simulink model "Zika_Model_continous"  (R2022b)
settings: Solver=ode4  StartTime=0.0  StopTime=275  FixedStep=0.01  RelTol=1e-3
values from neighbouring files (symbols this model uses):
  A_b_0 = 0    [Cibernetica_project.m]
  A_w_0 = 0    [Cibernetica_project.m]
  E_b_0 = 0    [Cibernetica_project.m]
  E_v_0 = 0    [Cibernetica_project.m]
  E_w_0 = 0    [Cibernetica_project.m]
  I_b_0 = 1    [Cibernetica_project.m]
  I_bm_0 = 0    [Cibernetica_project.m]
  I_v_0 = 1    [Cibernetica_project.m]
  I_w_0 = 1    [Cibernetica_project.m]
  I_wm_0 = 0    [Cibernetica_project.m]
  P = [alpha, rho_b, rho_w, beta_w, sigma_w, gamma_w, mu_w, pi_b, beta_b,      sigma_b, gamma_b, mu_b, pi_v, beta_v, b_v, sigma_v, mu_v, p, eta,      q_a, q_r, q_i, r]    [Cibernetica_project.m]
  R_b_0 = 0    [Cibernetica_project.m]
  R_w_0 = 0    [Cibernetica_project.m]
  S_b_0 = 8000    [Cibernetica_project.m]
  S_v_0 = 0.225*10^6    (= 225000)    [Cibernetica_project.m]
  S_w_0 = 8000    [Cibernetica_project.m]
settings Model: Creator=anton  LastModifiedBy=angel
settings SolverCC: EnableFixedStepZeroCrossing=on  MaxZcPerStep=10

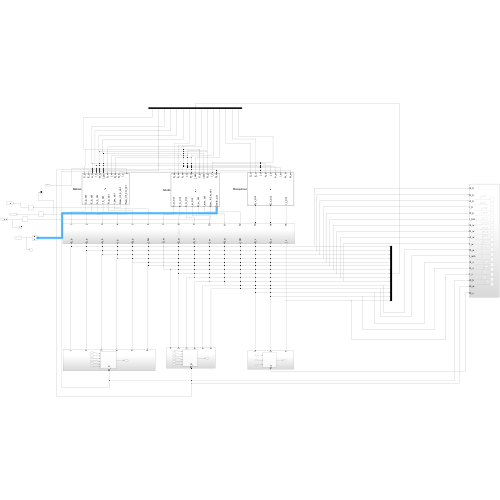
[thumbnail: Simulink's stored preview of the top-level diagram]
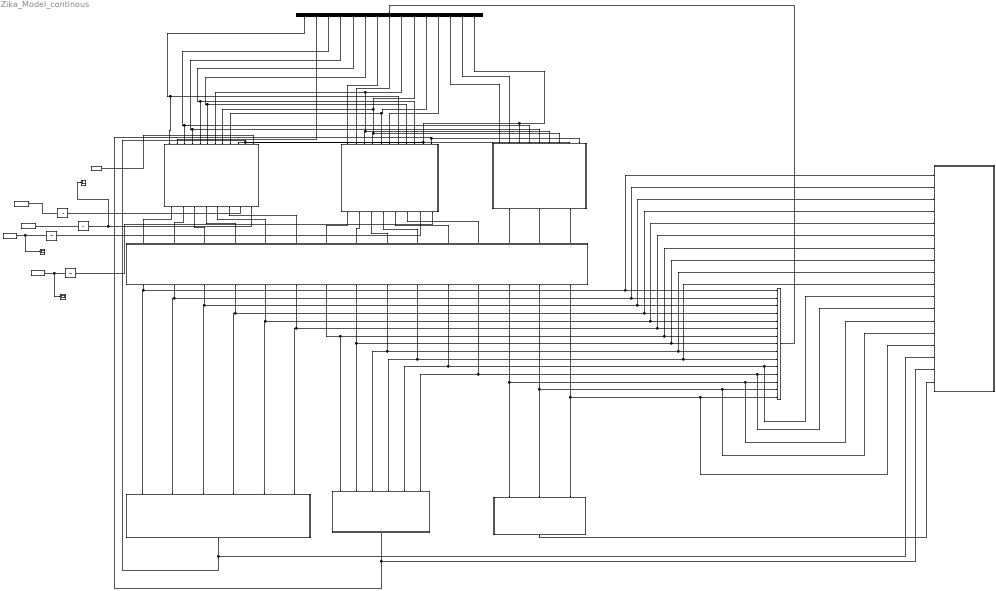
== system Zika_Model_continous ==
  Adults : MATLAB Function  TreatAsAtomicUnit=on  mask{P=P}
      mask prompts: P "Parametri del sistema"
  Babies : MATLAB Function  TreatAsAtomicUnit=on  mask{P=P}
      mask prompts: P "Parametri del sistema"
  Demux : Demux  Outputs=15
  Digital Clock : DigitalClock
  Integrator{,1..3} (4 alike) : Integrator
  Mosquitoes : MATLAB Function  TreatAsAtomicUnit=on  mask{P=P}
      mask prompts: P "Parametri del sistema"
  Mux : Mux  Inputs=15
  Scope : Scope
  Scope1 : Scope
  Scope2 : Scope
  Subsystem : Subsystem
  Subsystem1 : Subsystem
  Subsystem2 : Subsystem
  Subsystem3 : Subsystem
  Subsystem4 : Subsystem
  To Workspace : ToWorkspace  VariableName=New_inf_b  SampleTime=1
  To Workspace1 : ToWorkspace  VariableName=New_inf_w  SampleTime=1
  To Workspace2 : ToWorkspace  VariableName=New_inf_bm  SampleTime=1
  To Workspace3 : ToWorkspace  VariableName=Dead_Zika  SampleTime=1
  wires:
  Demux/5 -> Adults/9(R_b), Babies/5(R_b)
  Demux/6 -> Adults/8(I_bm), Babies/6(I_bm)
  Demux/9 -> Babies/7(A_w), Adults/3(A_w), Mosquitoes/6(A_w)
  Demux/4 -> Mosquitoes/5(I_b), Babies/4(I_b)
  Demux/7 -> Adults/1(S_w)
  Demux/2 -> Babies/2(E_b)
  Demux/11 -> Adults/5(R_w), Babies/9(R_w)
  Demux/15 -> Mosquitoes/3(I_v), Adults/10(I_v), Babies/11(I_v)
  Demux/14 -> Mosquitoes/2(E_v)
  Demux/8 -> Adults/2(E_w)
  Demux/13 -> Mosquitoes/1(S_v)
  Demux/10 -> Babies/8(I_w), Adults/4(I_w), Mosquitoes/7(I_w)
  Demux/12 -> Adults/6(I_wm)
  Subsystem2/1(N_v) -> Subsystem4/18(N_v)
  Demux/3 -> Mosquitoes/4(A_b), Babies/3(A_b)
  Demux/1 -> Babies/1(S_b), Adults/7(S_b)
  Mux/1 -> Demux/1
  Babies/1(S_b_dot) -> Subsystem3/1(In1)
  Babies/2(E_b_dot) -> Subsystem3/2(In2)
  Babies/3(A_b_dot) -> Subsystem3/3(In3)
  Babies/4(I_b_dot) -> Subsystem3/4(In4)
  Babies/5(R_b_dot) -> Subsystem3/5(In5)
  Babies/6(I_bm_dot) -> Subsystem3/6(In6)
  Adults/1(S_w_dot) -> Subsystem3/7(In7)
  Adults/2(E_w_dot) -> Subsystem3/8(In8)
  Adults/3(A_w_dot) -> Subsystem3/9(In9)
  Adults/4(I_w_dot) -> Subsystem3/10(In10)
  Adults/5(R_w_dot) -> Subsystem3/11(In11)
  Adults/6(I_wm_dot) -> Subsystem3/12(In12)
  Mosquitoes/1(S_v_dot) -> Subsystem3/13(In13)
  Mosquitoes/2(E_v_dot) -> Subsystem3/14(In14)
  Mosquitoes/3(I_v_dot) -> Subsystem3/15(In15)
  Subsystem3/1(S_b) -> Subsystem4/1(S_b), Mux/1, Subsystem/1(In1)
  Subsystem3/2(E_b) -> Subsystem4/2(E_b), Mux/2, Subsystem/2(In2)
  Subsystem3/3(A_b) -> Subsystem4/3(A_b), Mux/3, Subsystem/3(In3)
  Subsystem3/4(I_b) -> Subsystem4/4(I_b), Mux/4, Subsystem/4(In4)
  Subsystem3/5(R_b) -> Subsystem4/5(R_b), Mux/5, Subsystem/5(In5)
  Subsystem3/6(I_bm) -> Subsystem4/6(I_bm), Mux/6, Subsystem/6(In6)
  Subsystem3/7(S_w) -> Subsystem4/7(S_w), Mux/7, Subsystem1/1(In1)
  Subsystem3/8(E_w) -> Subsystem1/2(In2), Subsystem4/8(E_w), Mux/8
  Subsystem3/9(A_w) -> Subsystem1/3(In3), Subsystem4/9(A_w), Mux/9
  Subsystem3/10(I_w) -> Subsystem4/10(I_w), Mux/10, Subsystem1/4(In4)
  Subsystem3/11(R_w) -> Subsystem1/5(In5), Mux/11, Subsystem4/11(R_w)
  Subsystem3/12(I_wm) -> Subsystem4/12(I_wm), Mux/12, Subsystem1/6(In6)
  Subsystem3/13(S_v) -> Subsystem4/13(S_v), Mux/13, Subsystem2/1(In1)
  Subsystem3/15(I_v) -> Subsystem4/15(I_v), Mux/15, Subsystem2/3(In3)
  Subsystem3/14(E_v) -> Subsystem2/2(In2), Subsystem4/14(E_v), Mux/14
  Subsystem/1(N_b) -> Subsystem4/16(N_b), Mosquitoes/8(N_b), Babies/10(N_b)
  Subsystem1/1(N_w) -> Subsystem4/17(N_w), Mosquitoes/9(N_w), Adults/11(N_w)
  Babies/7(New_inf_b_dot) -> Integrator/1
  Integrator/1 -> To Workspace/1
  Integrator1/1 -> Scope1/1, To Workspace1/1
  Adults/7(New_Inf_w_dot) -> Integrator1/1
  Integrator2/1 -> To Workspace2/1
  Babies/8(New_inf_bm_dot) -> Scope/1, Integrator2/1
  Digital Clock/1 -> Babies/12(t)
  Integrator3/1 -> Scope2/1, To Workspace3/1
  Adults/8(Death_dot) -> Integrator3/1

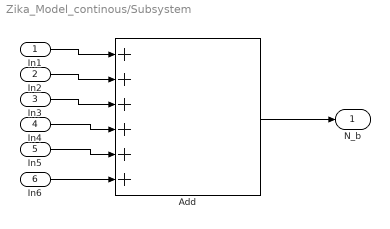
== system Zika_Model_continous/Subsystem ==
  In1 : Inport
  In2 : Inport  Port=2
  In3 : Inport  Port=3
  In4 : Inport  Port=4
  In5 : Inport  Port=5
  In6 : Inport  Port=6
  Add : Sum  Inputs=++++++
  N_b : Outport
  wires:
  In2/1 -> Add/2
  Add/1 -> N_b/1
  In1/1 -> Add/1
  In6/1 -> Add/6
  In5/1 -> Add/5
  In4/1 -> Add/4
  In3/1 -> Add/3

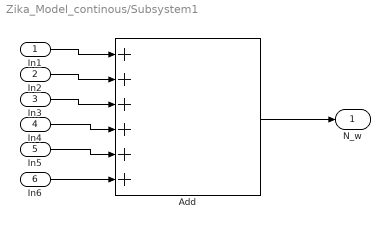
== system Zika_Model_continous/Subsystem1 ==
  In1 : Inport
  In2 : Inport  Port=2
  In3 : Inport  Port=3
  In4 : Inport  Port=4
  In5 : Inport  Port=5
  In6 : Inport  Port=6
  Add : Sum  Inputs=++++++
  N_w : Outport
  wires:
  In2/1 -> Add/2
  Add/1 -> N_w/1
  In1/1 -> Add/1
  In6/1 -> Add/6
  In5/1 -> Add/5
  In4/1 -> Add/4
  In3/1 -> Add/3

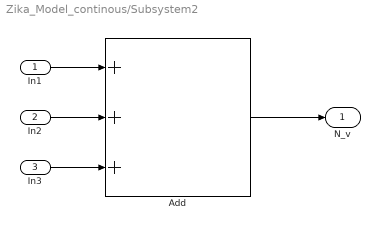
== system Zika_Model_continous/Subsystem2 ==
  In1 : Inport
  In2 : Inport  Port=2
  In3 : Inport  Port=3
  Add : Sum  Inputs=+++
  N_v : Outport
  wires:
  In2/1 -> Add/2
  Add/1 -> N_v/1
  In1/1 -> Add/1
  In3/1 -> Add/3

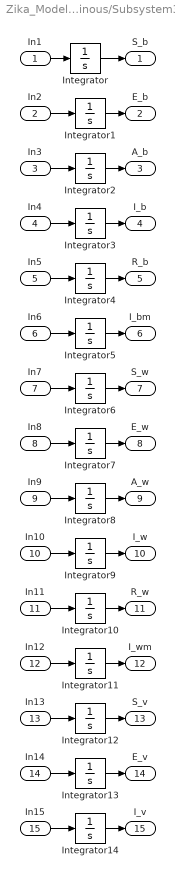
== system Zika_Model_continous/Subsystem3 ==
  In1 : Inport
  In2 : Inport  Port=2
  In3 : Inport  Port=3
  In4 : Inport  Port=4
  In5 : Inport  Port=5
  In6 : Inport  Port=6
  In7 : Inport  Port=7
  In8 : Inport  Port=8
  In9 : Inport  Port=9
  In10 : Inport  Port=10
  In11 : Inport  Port=11
  In12 : Inport  Port=12
  In13 : Inport  Port=13
  In14 : Inport  Port=14
  In15 : Inport  Port=15
  Integrator : Integrator  InitialCondition=S_b_0  ContinuousStateAttributes='S_b'
  Integrator1 : Integrator  InitialCondition=E_b_0  ContinuousStateAttributes='E_b'
  Integrator10 : Integrator  InitialCondition=R_w_0  ContinuousStateAttributes='R_w'
  Integrator11 : Integrator  InitialCondition=I_wm_0  ContinuousStateAttributes='I_wm'
  Integrator12 : Integrator  InitialCondition=S_v_0  ContinuousStateAttributes='S_v'
  Integrator13 : Integrator  InitialCondition=E_v_0  ContinuousStateAttributes='E_v'
  Integrator14 : Integrator  InitialCondition=I_v_0  ContinuousStateAttributes='I_v'
  Integrator2 : Integrator  InitialCondition=A_b_0  ContinuousStateAttributes='A_b'
  Integrator3 : Integrator  InitialCondition=I_b_0  ContinuousStateAttributes='I_b'
  Integrator4 : Integrator  InitialCondition=R_b_0  ContinuousStateAttributes='R_b'
  Integrator5 : Integrator  InitialCondition=I_bm_0  ContinuousStateAttributes='I_bm'
  Integrator6 : Integrator  InitialCondition=S_w_0  ContinuousStateAttributes='S_w'
  Integrator7 : Integrator  InitialCondition=E_w_0  ContinuousStateAttributes='E_w'
  Integrator8 : Integrator  InitialCondition=A_w_0  ContinuousStateAttributes='A_w'
  Integrator9 : Integrator  InitialCondition=I_w_0  ContinuousStateAttributes='I_w'
  S_b : Outport
  E_b : Outport  Port=2
  A_b : Outport  Port=3
  I_b : Outport  Port=4
  R_b : Outport  Port=5
  I_bm : Outport  Port=6
  S_w : Outport  Port=7
  E_w : Outport  Port=8
  A_w : Outport  Port=9
  I_w : Outport  Port=10
  R_w : Outport  Port=11
  I_wm : Outport  Port=12
  S_v : Outport  Port=13
  E_v : Outport  Port=14
  I_v : Outport  Port=15
  wires:
  In9/1 -> Integrator8/1
  In1/1 -> Integrator/1
  In12/1 -> Integrator11/1
  Integrator/1 -> S_b/1
  In2/1 -> Integrator1/1
  Integrator12/1 -> S_v/1
  Integrator13/1 -> E_v/1
  In13/1 -> Integrator12/1
  Integrator2/1 -> A_b/1
  Integrator1/1 -> E_b/1
  In6/1 -> Integrator5/1
  In14/1 -> Integrator13/1
  Integrator9/1 -> I_w/1
  Integrator4/1 -> R_b/1
  In11/1 -> Integrator10/1
  In3/1 -> Integrator2/1
  Integrator5/1 -> I_bm/1
  Integrator11/1 -> I_wm/1
  Integrator7/1 -> E_w/1
  Integrator14/1 -> I_v/1
  Integrator10/1 -> R_w/1
  In4/1 -> Integrator3/1
  Integrator3/1 -> I_b/1
  Integrator6/1 -> S_w/1
  In15/1 -> Integrator14/1
  Integrator8/1 -> A_w/1
  In10/1 -> Integrator9/1
  In5/1 -> Integrator4/1
  In7/1 -> Integrator6/1
  In8/1 -> Integrator7/1

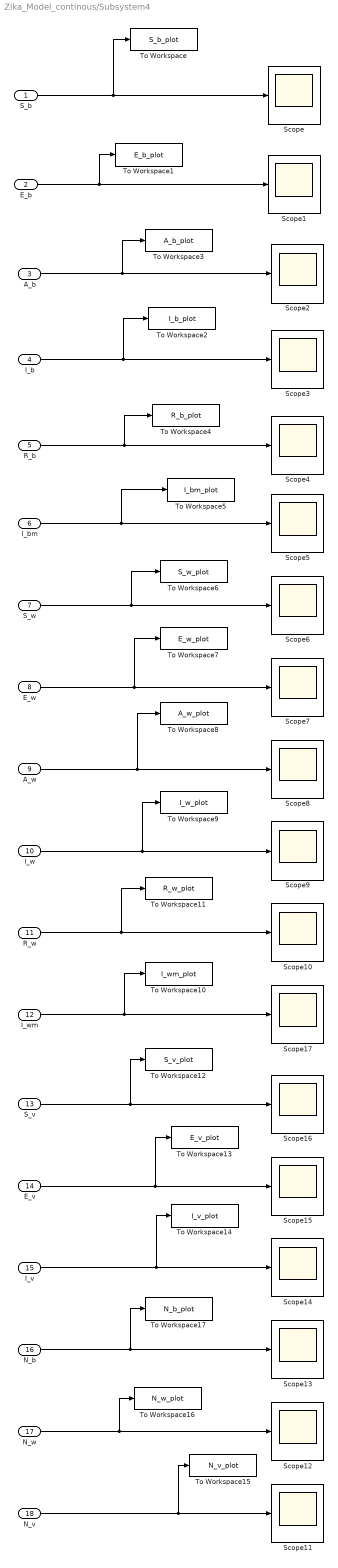
== system Zika_Model_continous/Subsystem4 ==
  S_b : Inport
  E_b : Inport  Port=2
  A_b : Inport  Port=3
  I_b : Inport  Port=4
  R_b : Inport  Port=5
  I_bm : Inport  Port=6
  S_w : Inport  Port=7
  E_w : Inport  Port=8
  A_w : Inport  Port=9
  I_w : Inport  Port=10
  R_w : Inport  Port=11
  I_wm : Inport  Port=12
  S_v : Inport  Port=13
  E_v : Inport  Port=14
  I_v : Inport  Port=15
  N_b : Inport  Port=16
  N_w : Inport  Port=17
  N_v : Inport  Port=18
  Scope{,1..17} (18 alike) : Scope
  To Workspace : ToWorkspace  VariableName=S_b_plot  SampleTime=1
  To Workspace1 : ToWorkspace  VariableName=E_b_plot  SampleTime=1
  To Workspace10 : ToWorkspace  VariableName=I_wm_plot  SampleTime=1
  To Workspace11 : ToWorkspace  VariableName=R_w_plot  SampleTime=1
  To Workspace12 : ToWorkspace  VariableName=S_v_plot  SampleTime=1
  To Workspace13 : ToWorkspace  VariableName=E_v_plot  SampleTime=1
  To Workspace14 : ToWorkspace  VariableName=I_v_plot  SampleTime=1
  To Workspace15 : ToWorkspace  VariableName=N_v_plot  SampleTime=1
  To Workspace16 : ToWorkspace  VariableName=N_w_plot  SampleTime=1
  To Workspace17 : ToWorkspace  VariableName=N_b_plot  SampleTime=1
  To Workspace2 : ToWorkspace  VariableName=I_b_plot  SampleTime=1
  To Workspace3 : ToWorkspace  VariableName=A_b_plot  SampleTime=1
  To Workspace4 : ToWorkspace  VariableName=R_b_plot  SampleTime=1
  To Workspace5 : ToWorkspace  VariableName=I_bm_plot  SampleTime=1
  To Workspace6 : ToWorkspace  VariableName=S_w_plot  SampleTime=1
  To Workspace7 : ToWorkspace  VariableName=E_w_plot  SampleTime=1
  To Workspace8 : ToWorkspace  VariableName=A_w_plot  SampleTime=1
  To Workspace9 : ToWorkspace  VariableName=I_w_plot  SampleTime=1
  wires:
  E_w/1 -> To Workspace7/1, Scope7/1
  E_b/1 -> To Workspace1/1, Scope1/1
  R_w/1 -> To Workspace11/1, Scope10/1
  A_b/1 -> To Workspace3/1, Scope2/1
  A_w/1 -> To Workspace8/1, Scope8/1
  R_b/1 -> To Workspace4/1, Scope4/1
  I_w/1 -> To Workspace9/1, Scope9/1
  S_v/1 -> To Workspace12/1, Scope16/1
  S_b/1 -> To Workspace/1, Scope/1
  I_wm/1 -> To Workspace10/1, Scope17/1
  I_bm/1 -> To Workspace5/1, Scope5/1
  I_b/1 -> To Workspace2/1, Scope3/1
  S_w/1 -> To Workspace6/1, Scope6/1
  E_v/1 -> To Workspace13/1, Scope15/1
  I_v/1 -> To Workspace14/1, Scope14/1
  N_v/1 -> To Workspace15/1, Scope11/1
  N_w/1 -> To Workspace16/1, Scope12/1
  N_b/1 -> To Workspace17/1, Scope13/1

== matlab function Zika_Model_continous/Adults ==
  data: S_w input; E_w input; A_w input; I_w input; R_w input; I_wm input; S_b input; S_w_dot output; I_bm input; R_b input; I_v input; N_w input; E_w_dot output; A_w_dot output; I_w_dot output; R_w_dot output; I_wm_dot output; P parameter; New_Inf_w_dot output; Death_dot output
function [S_w_dot, E_w_dot, A_w_dot, I_w_dot, R_w_dot, I_wm_dot, New_Inf_w_dot, Death_dot] = Adults(S_w,...
    E_w, A_w, I_w, R_w, I_wm, S_b, I_bm, R_b, I_v, N_w, P)

alpha = P(1);
rho_b = P(2);
rho_w = P(3);
beta_w = P(4);
sigma_w = P(5);
gamma_w = P(6);
mu_w = P(7);
pi_b = P(8);
beta_b = P(9);
sigma_b =  P(10);
gamma_b = P(11);
mu_b =  P(12);
pi_v =  P(13);
beta_v = P(14);
b_v = P(15);
sigma_v = P(16);
mu_v = P(17);
p = P(18);
eta = P(19);
q_a = P(20);
q_r = P(21);
q_i = P(22);
r = P(23);


lambda_w = (beta_w*b_v*I_v)/N_w;

S_w_dot = alpha*S_b - lambda_w*S_w - mu_w*S_w;
E_w_dot = lambda_w*S_w - (sigma_w + mu_v)*E_w;
A_w_dot = (1-p)*sigma_w*E_w - (gamma_w + mu_w)*A_w;
I_w_dot = p*sigma_w*E_w - (gamma_w + mu_w)*I_w;
I_wm_dot = alpha*I_bm - mu_w*I_wm;
R_w_dot = alpha*R_b + gamma_w*A_w + gamma_w*I_w - mu_w*R_w;

New_Inf_w_dot = sigma_w*E_w;
Death_dot = mu_w*(S_w + E_w + I_w + I_wm + R_w);

== matlab function Zika_Model_continous/Babies ==
  data: S_b input; S_b_dot output; E_b input; A_b input; I_b input; R_b input; I_bm input; E_b_dot output; A_b_dot output; I_b_dot output; R_b_dot output; I_bm_dot output; A_w input; I_w input; R_w input; P parameter; N_b input; I_v input; New_inf_b_dot output; New_inf_bm_dot output; t input
function [S_b_dot, E_b_dot, A_b_dot, I_b_dot, R_b_dot, I_bm_dot,New_inf_b_dot, New_inf_bm_dot] = Babies( ... 
    S_b, E_b, A_b, I_b, R_b, I_bm, A_w, I_w, R_w, P, N_b, I_v,t)
alpha = P(1);
rho_b = P(2);
rho_w = P(3);
beta_w = P(4);
sigma_w = P(5);
gamma_w = P(6);
mu_w = P(7);
pi_b = P(8);
beta_b = P(9);
sigma_b =  P(10);
gamma_b = P(11);
mu_b =  P(12);
pi_v =  P(13);
beta_v = P(14);
b_v = P(15);
sigma_v = P(16);
mu_v = P(17);
p = P(18);
eta = P(19);
q_a = P(20);
q_r = P(21);
q_i = P(22);
r = P(23);

if S_b > 0
    is_notzero = 1;
else
    is_notzero = 0;
end

lambda_b = (eta*beta_b*b_v*I_v)/N_b;

S_b_dot = pi_b - is_notzero*q_a*pi_b*A_w - is_notzero*q_i*pi_b*I_w...
    - is_notzero*q_r*pi_b*R_w - is_notzero*lambda_b*S_b -... 
    is_notzero*(alpha + mu_b)*S_b;
A_b_dot = is_notzero*q_a*pi_b*A_w + (1 - p)*sigma_b*E_b - (alpha + gamma_b + mu_b)*A_b;
I_b_dot = is_notzero*q_i*pi_b*I_w + p*sigma_b*E_b - (alpha +gamma_b + mu_b)*I_b;
I_bm_dot = is_notzero*r*q_r*pi_b*R_w - (alpha + mu_b)*I_bm;
R_b_dot = is_notzero*(1-r)*q_r*pi_b*R_w + gamma_b*A_b + gamma_b*I_b - (alpha + mu_b)*R_b;
E_b_dot = lambda_b*S_b - (alpha + sigma_b + mu_b)*E_b;

New_inf_b_dot = is_notzero*q_a*pi_b*A_w + sigma_b*E_b + is_notzero*q_i*pi_b*I_w;
New_inf_bm_dot = is_notzero*r*q_r*pi_b*R_w;

== matlab function Zika_Model_continous/Mosquitoes ==
  data: S_v input; E_v input; I_v input; S_v_dot output; A_b input; I_b input; A_w input; I_w input; N_b input; N_w input; E_v_dot output; I_v_dot output; P parameter
function [S_v_dot, E_v_dot, I_v_dot] = Mosquitoes(S_v, E_v, I_v, ... 
    A_b, I_b, A_w, I_w, N_b, N_w, P)

alpha = P(1);
rho_b = P(2);
rho_w = P(3);
beta_w = P(4);
sigma_w = P(5);
gamma_w = P(6);
mu_w = P(7);
pi_b = P(8);
beta_b = P(9);
sigma_b =  P(10);
gamma_b = P(11);
mu_b =  P(12);
pi_v =  P(13);
beta_v = P(14);
b_v = P(15);
sigma_v = P(16);
mu_v = P(17);
p = P(18);
eta = P(19);
q_a = P(20);
q_r = P(21);
q_i = P(22);
r = P(23);

lambda_v = beta_v*b_v*((I_w + rho_w*A_w + eta*(I_b + rho_b*A_b))/ ...
    (N_w + eta*N_b));

S_v_dot = pi_v - lambda_v*S_v - mu_v*S_v;
E_v_dot = lambda_v*S_v - (mu_v + sigma_v)*E_v;
I_v_dot = sigma_v*E_v - mu_v*I_v;
